simulink model "amisa"  (R2013a)
settings: Solver=VariableStepDiscrete  SolverMode=SingleTasking  StartTime=0.0  StopTime=5000  RelTol=1e-3
undefined symbols (not defined in the file or in its folder): gcbh, sfp, xlBlockLoadCallback
libraries: xbsIndex_r4 x4683, dspsigops x32, xps_library x30, casper_library_misc x27, casper_library_delays x2
(part 8 of 43)

== system amisa/gpio_switch_states ==
  addr : Inport
  data_in : Inport  Port=2
  we : Inport  Port=3
  amisa_gpio_switch_states_addr : xbsIndex_r4/Gateway Out  inherit_from_input=off  hdl_port=on  timing_constraint=None  locs_specified=off  LOCs={'A5','B9','A9','C1','A3','G6','E9','A6','A7','A8','B8','B1','B3','D9','B5','B4','B6','C2'}  UseAsDAC=off  DACChannel='1'  block_type=gatewayout
      settings: infoedit="Gateway out block.  Converts Xilinx fixed point inputs into ouputs of type Simulink integer, double, or fixed point.<P><P>Hardware notes:  In hardware these blocks become top level output ports or are discarded, depending on how they are configured."  xl_area=[0, 0, 0, 0, 0, 0, 0]  sginterface={'Nallatech'=>{'xdspkit'=>{'non_memory_mapped_port'=>'uprev_Shared_BRAM_addr'}},'Xilinx'=>{'jtaghwcosim'=>{'non_memory_mapped_port'=>'uprev_Shared_BRAM_addr'},'xdspkit'=>{'non_memory_mapped_port'=>'uprev_Shared_BRAM_addr'}}}
  amisa_gpio_switch_states_data_in : xbsIndex_r4/Gateway Out  inherit_from_input=off  hdl_port=on  timing_constraint=None  locs_specified=off  LOCs={'B21','B22','A22','B23','B19','C19','A20','A21','A23','B24','A24','A25','E18','D18','C18','B18'}  UseAsDAC=off  DACChannel='1'  block_type=gatewayout
      settings: infoedit="Gateway out block.  Converts Xilinx fixed point inputs into ouputs of type Simulink integer, double, or fixed point.<P><P>Hardware notes:  In hardware these blocks become top level output ports or are discarded, depending on how they are configured."  xl_area=[0, 0, 0, 0, 0, 0, 0]  sginterface={'Nallatech'=>{'xdspkit'=>{'non_memory_mapped_port'=>'uprev_Shared_BRAM_data_in'}},'Xilinx'=>{'jtaghwcosim'=>{'non_memory_mapped_port'=>'uprev_Shared_BRAM_data_in'},'xdspkit'=>{'non_memory_mapped_port'=>'uprev_Shared_BRAM_data_in'}}}
  amisa_gpio_switch_states_data_out : xbsIndex_r4/Gateway In  gui_display_data_type=Fixed-point  arith_type=Unsigned  n_bits=8  bin_pt=0  preci_type=Single  exp_width=8  frac_width=24  quantization=Truncate  overflow=Wrap  period=sample_rate  dbl_ovrd=off  timing_constraint=None  locs_specified=off  LOCs={}  UseAsADC=off  ADCChannel='1'  inherit_from_input=off  hdl_port=on  block_type=gatewayin
      settings: xl_area=[0, 0, 0, 0, 0, 0, 0]
  amisa_gpio_switch_states_we : xbsIndex_r4/Gateway Out  inherit_from_input=off  hdl_port=on  timing_constraint=None  locs_specified=off  LOCs={'A14'}  UseAsDAC=off  DACChannel='1'  block_type=gatewayout
      settings: infoedit="Gateway out block.  Converts Xilinx fixed point inputs into ouputs of type Simulink integer, double, or fixed point.<P><P>Hardware notes:  In hardware these blocks become top level output ports or are discarded, depending on how they are configured."  xl_area=[0, 0, 0, 0, 0, 0, 0]
  calc_add : Subsystem  mask{data_width=8, addr_width=12, sample_rate=sample_rate}
      mask prompts: data_width "data width"; addr_width "address width"; sample_rate "sample rate"
  convert_addr : xbsIndex_r4/Convert  gui_display_data_type=Fixed-point  arith_type=Unsigned  n_bits=addr_width  bin_pt=0  float_type=Single  exp_bits=8  fraction_bits=24  quantization=Truncate  overflow=Wrap  en=off  latency=0  dbl_ovrd=off  pipeline=off  block_type=convert
      settings: xl_area=[0, 0, 0, 0, 0, 0, 0]
  convert_din1 : xbsIndex_r4/Convert  gui_display_data_type=Fixed-point  arith_type=Unsigned  n_bits=8  bin_pt=0  float_type=Single  exp_bits=8  fraction_bits=24  quantization=Truncate  overflow=Wrap  en=off  latency=0  dbl_ovrd=off  pipeline=off  block_type=convert
      settings: xl_area=[0, 0, 0, 0, 0, 0, 0]
  convert_we : xbsIndex_r4/Convert  gui_display_data_type=Fixed-point  arith_type=Unsigned  n_bits=1  bin_pt=0  float_type=Single  exp_bits=8  fraction_bits=24  quantization=Truncate  overflow=Wrap  en=off  latency=0  dbl_ovrd=off  pipeline=off  block_type=convert
      settings: xl_area=[0, 0, 0, 0, 0, 0, 0]
  mem : Subsystem
  munge_in : Subsystem  AncestorBlock=casper_library_flow_control/munge  mask(munge){divisions=1, div_size=8, order=[0], arith_type_out=Unsigned, bin_pt_out=0}
      mask prompts: divisions "Number of divisions"; div_size "Division size (bits)"; order "Division packing order"; arith_type_out "Output arithmetic type"; bin_pt_out "Output binary point"
      mask help: Splits an input bus into the specified number of divisions and then recombines them in the order specified (most significant division = 0,least = number divisions-1)
      mask init:
      | munge_init(gcb, ...
      |     'divisions', divisions, ...
      |     'div_size', div_size, ...
      |     'order', order, ...
      |     'arith_type_out', arith_type_out, ...
      |     'bin_pt_out', bin_pt_out);
      settings: AttributesFormatString=|
      | split:8
      | join:0
      | Unsigned [8,0]
      mask TypeOptions arith_type_out: Unsigned | Signed  (2's comp) | Floating-point
  munge_out : Subsystem  AncestorBlock=casper_library_flow_control/munge  mask(munge){divisions=1, div_size=8, order=[0], arith_type_out=Unsigned, bin_pt_out=0}
      mask prompts: divisions "Number of divisions"; div_size "Division size (bits)"; order "Division packing order"; arith_type_out "Output arithmetic type"; bin_pt_out "Output binary point"
      mask help: Splits an input bus into the specified number of divisions and then recombines them in the order specified (most significant division = 0,least = number divisions-1)
      mask init:
      | munge_init(gcb, ...
      |     'divisions', divisions, ...
      |     'div_size', div_size, ...
      |     'order', order, ...
      |     'arith_type_out', arith_type_out, ...
      |     'bin_pt_out', bin_pt_out);
      settings: AttributesFormatString=|
      | split:8
      | join:0
      | Unsigned [8,0]
      mask TypeOptions arith_type_out: Unsigned | Signed  (2's comp) | Floating-point
  data_out : Outport
  wires:
  convert_addr/1 -> amisa_gpio_switch_states_addr/1
  convert_din1/1 -> amisa_gpio_switch_states_data_in/1
  data_in/1 -> munge_in/1(din)
  calc_add/1(out) -> convert_addr/1
  amisa_gpio_switch_states_we/1 -> mem/3(In3)
  amisa_gpio_switch_states_data_in/1 -> mem/2(In2)
  amisa_gpio_switch_states_addr/1 -> mem/1(In1)
  convert_we/1 -> amisa_gpio_switch_states_we/1
  amisa_gpio_switch_states_data_out/1 -> munge_out/1(din)
  mem/1(Out1) -> amisa_gpio_switch_states_data_out/1
  addr/1 -> calc_add/1(in)
  we/1 -> convert_we/1
  munge_out/1(dout) -> data_out/1
  munge_in/1(dout) -> convert_din1/1

== system amisa/ip_base ==
  sim_1 : Inport
  amisa_ip_base_user_data_out : xbsIndex_r4/Gateway In  gui_display_data_type=Fixed-point  arith_type=Unsigned  n_bits=32  bin_pt=0  preci_type=Single  exp_width=8  frac_width=24  quantization="Round  (unbiased: +/- Inf)"  overflow=Saturate  period=1  dbl_ovrd=off  timing_constraint=None  locs_specified=off  LOCs={}  UseAsADC=off  ADCChannel='1'  inherit_from_input=off  hdl_port=on  block_type=gatewayin
  io_delay : xbsIndex_r4/Delay  rst=off  infoeditControl=Selection of Reset will increase slice count due to use of real FFs and instead of SRLs  en=off  latency=0  dbl_ovrd=off  reg_retiming=on  block_type=delay
  reint1 : xbsIndex_r4/Reinterpret  force_arith_type=on  arith_type=Unsigned  force_bin_pt=on  bin_pt=0  block_type=reinterpret
  slice_reg : xbsIndex_r4/Slice  nbits=32  boolean_output=off  mode=Lower Bit Location + Width  bit1=0  base1=MSB of Input  bit0=0  base0=LSB of Input  dbl_ovrd=off  block_type=slice
  in_reg : Outport
  wires:
  amisa_ip_base_user_data_out/1 -> io_delay/1
  sim_1/1 -> amisa_ip_base_user_data_out/1
  io_delay/1 -> slice_reg/1
  slice_reg/1 -> reint1/1
  reint1/1 -> in_reg/1

== system amisa/leds ==
  warning : Inport
  rst : Inport  Port=2
  sync_led : Inport  Port=3
  pps : Inport  Port=4
  comms : Inport  Port=5
  ps_gpio : Inport  Port=6
  noise_gpio : Inport  Port=7
  or0 : Inport  Port=8
  or1 : Inport  Port=9
  0 : xps_library/gpio  Tag=xps:gpio  io_group=ROACH2:led  io_dir=out  arith_type=Boolean  bitwidth=1  bin_pt=0  bit_index=0  sample_period=1  use_single_ended=off  use_ddr=off  reg_iob=on  reg_clk_phase=0  termination=None
      link override convert: arith_type=Boolean  n_bits=1  bin_pt=0
  1 : xps_library/gpio  Tag=xps:gpio  io_group=ROACH2:led  io_dir=out  arith_type=Boolean  bitwidth=1  bin_pt=0  bit_index=1  sample_period=1  use_single_ended=off  use_ddr=off  reg_iob=on  reg_clk_phase=0  termination=None
      link override convert: arith_type=Boolean  n_bits=1  bin_pt=0
  2 : xps_library/gpio  Tag=xps:gpio  io_group=ROACH2:led  io_dir=out  arith_type=Boolean  bitwidth=1  bin_pt=0  bit_index=2  sample_period=1  use_single_ended=off  use_ddr=off  reg_iob=on  reg_clk_phase=0  termination=None
      link override convert: arith_type=Boolean  n_bits=1  bin_pt=0
  3 : xps_library/gpio  Tag=xps:gpio  io_group=ROACH2:led  io_dir=out  arith_type=Boolean  bitwidth=1  bin_pt=0  bit_index=3  sample_period=1  use_single_ended=off  use_ddr=off  reg_iob=on  reg_clk_phase=0  termination=None
      link override convert: arith_type=Boolean  n_bits=1  bin_pt=0
  4 : xps_library/gpio  Tag=xps:gpio  io_group=ROACH2:led  io_dir=out  arith_type=Boolean  bitwidth=1  bin_pt=0  bit_index=4  sample_period=1  use_single_ended=off  use_ddr=off  reg_iob=on  reg_clk_phase=0  termination=None
      link override convert: arith_type=Boolean  n_bits=1  bin_pt=0
  5 : xps_library/gpio  Tag=xps:gpio  io_group=ROACH2:led  io_dir=out  arith_type=Boolean  bitwidth=1  bin_pt=0  bit_index=5  sample_period=1  use_single_ended=off  use_ddr=off  reg_iob=on  reg_clk_phase=0  termination=None
      link override convert: arith_type=Boolean  n_bits=1  bin_pt=0
  6 : xps_library/gpio  Tag=xps:gpio  io_group=ROACH2:led  io_dir=out  arith_type=Boolean  bitwidth=1  bin_pt=0  bit_index=6  sample_period=1  use_single_ended=off  use_ddr=off  reg_iob=on  reg_clk_phase=0  termination=None
      link override convert: arith_type=Boolean  n_bits=1  bin_pt=0
  7 : xps_library/gpio  Tag=xps:gpio  io_group=ROACH2:led  io_dir=out  arith_type=Boolean  bitwidth=1  bin_pt=0  bit_index=7  sample_period=1  use_single_ended=off  use_ddr=off  reg_iob=on  reg_clk_phase=0  termination=None
      link override convert: arith_type=Boolean  n_bits=1  bin_pt=0
  Counter1 : xbsIndex_r4/Counter  cnt_type=Free Running  cnt_to=Inf  operation=Up  start_count=0  cnt_by_val=1  arith_type=Unsigned  n_bits=1  bin_pt=0  load_pin=off  rst=on  en=on  explicit_period=on  period=1  dbl_ovrd=off  use_behavioral_HDL=off  implementation=Fabric  use_rpm=off  block_type=counter
  Counter2 : xbsIndex_r4/Counter  cnt_type=Free Running  cnt_to=Inf  operation=Up  start_count=0  cnt_by_val=1  arith_type=Unsigned  n_bits=1  bin_pt=0  load_pin=off  rst=on  en=on  explicit_period=on  period=1  dbl_ovrd=off  use_behavioral_HDL=off  implementation=Fabric  use_rpm=off  block_type=counter
  Logical2 : xbsIndex_r4/Logical  logical_function=OR  inputs=3  en=off  latency=1  precision=Full  arith_type=Unsigned  n_bits=16  bin_pt=0  align_bp=on  dbl_ovrd=off  block_type=logical
      settings: block_version=11.4
  Logical{3..6} (4 alike) : xbsIndex_r4/Logical  logical_function=OR  inputs=2  en=off  latency=1  precision=Full  arith_type=Unsigned  n_bits=16  bin_pt=0  align_bp=on  dbl_ovrd=off  block_type=logical
      settings: block_version=11.4
  Slice{,1..3} (4 alike) : xbsIndex_r4/Slice  nbits=1  boolean_output=on  mode=Upper Bit Location + Width  bit1=0  base1=MSB of Input  bit0=0  base0=LSB of Input  dbl_ovrd=off  block_type=slice
  Terminator{5..8,10..13} (8 alike) : Terminator
  pipeline : Subsystem  AncestorBlock=casper_library_delays/pipeline  mask(pipeline){latency=3}
      mask help:
      | An explicitly laid-out delay line to avoid mapping to SRL16s
      | for use in pipelining to help achieve timing closure.
      mask init:
      | pipeline_init(gcb,'latency',latency);
      settings: AttributesFormatString=Latency = %<latency>
      mask Display:
      | port_label('input', 1, 'd');
      | port_label('output', 1, 'q');
      | disp(['Z^-', num2str(latency)]);
  pipeline1 : Subsystem  AncestorBlock=casper_library_delays/pipeline  mask(pipeline){latency=3}
      mask help:
      | An explicitly laid-out delay line to avoid mapping to SRL16s
      | for use in pipelining to help achieve timing closure.
      mask init:
      | pipeline_init(gcb,'latency',latency);
      settings: AttributesFormatString=Latency = %<latency>
      mask Display:
      | port_label('input', 1, 'd');
      | port_label('output', 1, 'q');
      | disp(['Z^-', num2str(latency)]);
  pipeline12 : Subsystem  AncestorBlock=casper_library_delays/pipeline  mask(pipeline){latency=2}
      mask help:
      | An explicitly laid-out delay line to avoid mapping to SRL16s
      | for use in pipelining to help achieve timing closure.
      mask init:
      | pipeline_init(gcb,'latency',latency);
      settings: AttributesFormatString=Latency = %<latency>
      mask Display:
      | port_label('input', 1, 'd');
      | port_label('output', 1, 'q');
      | disp(['Z^-', num2str(latency)]);
  pipeline13 : Subsystem  AncestorBlock=casper_library_delays/pipeline  mask(pipeline){latency=2}
      mask help:
      | An explicitly laid-out delay line to avoid mapping to SRL16s
      | for use in pipelining to help achieve timing closure.
      mask init:
      | pipeline_init(gcb,'latency',latency);
      settings: AttributesFormatString=Latency = %<latency>
      mask Display:
      | port_label('input', 1, 'd');
      | port_label('output', 1, 'q');
      | disp(['Z^-', num2str(latency)]);
  pipeline14 : Subsystem  AncestorBlock=casper_library_delays/pipeline  mask(pipeline){latency=2}
      mask help:
      | An explicitly laid-out delay line to avoid mapping to SRL16s
      | for use in pipelining to help achieve timing closure.
      mask init:
      | pipeline_init(gcb,'latency',latency);
      settings: AttributesFormatString=Latency = %<latency>
      mask Display:
      | port_label('input', 1, 'd');
      | port_label('output', 1, 'q');
      | disp(['Z^-', num2str(latency)]);
  pipeline2 : Subsystem  AncestorBlock=casper_library_delays/pipeline  mask(pipeline){latency=3}
      mask help:
      | An explicitly laid-out delay line to avoid mapping to SRL16s
      | for use in pipelining to help achieve timing closure.
      mask init:
      | pipeline_init(gcb,'latency',latency);
      settings: AttributesFormatString=Latency = %<latency>
      mask Display:
      | port_label('input', 1, 'd');
      | port_label('output', 1, 'q');
      | disp(['Z^-', num2str(latency)]);
  pipeline3 : Subsystem  AncestorBlock=casper_library_delays/pipeline  mask(pipeline){latency=3}
      mask help:
      | An explicitly laid-out delay line to avoid mapping to SRL16s
      | for use in pipelining to help achieve timing closure.
      mask init:
      | pipeline_init(gcb,'latency',latency);
      settings: AttributesFormatString=Latency = %<latency>
      mask Display:
      | port_label('input', 1, 'd');
      | port_label('output', 1, 'q');
      | disp(['Z^-', num2str(latency)]);
  pipeline4 : Subsystem  AncestorBlock=casper_library_delays/pipeline  mask(pipeline){latency=3}
      mask help:
      | An explicitly laid-out delay line to avoid mapping to SRL16s
      | for use in pipelining to help achieve timing closure.
      mask init:
      | pipeline_init(gcb,'latency',latency);
      settings: AttributesFormatString=Latency = %<latency>
      mask Display:
      | port_label('input', 1, 'd');
      | port_label('output', 1, 'q');
      | disp(['Z^-', num2str(latency)]);
  pipeline5 : Subsystem  AncestorBlock=casper_library_delays/pipeline  mask(pipeline){latency=3}
      mask help:
      | An explicitly laid-out delay line to avoid mapping to SRL16s
      | for use in pipelining to help achieve timing closure.
      mask init:
      | pipeline_init(gcb,'latency',latency);
      settings: AttributesFormatString=Latency = %<latency>
      mask Display:
      | port_label('input', 1, 'd');
      | port_label('output', 1, 'q');
      | disp(['Z^-', num2str(latency)]);
  pipeline6 : Subsystem  AncestorBlock=casper_library_delays/pipeline  mask(pipeline){latency=3}
      mask help:
      | An explicitly laid-out delay line to avoid mapping to SRL16s
      | for use in pipelining to help achieve timing closure.
      mask init:
      | pipeline_init(gcb,'latency',latency);
      settings: AttributesFormatString=Latency = %<latency>
      mask Display:
      | port_label('input', 1, 'd');
      | port_label('output', 1, 'q');
      | disp(['Z^-', num2str(latency)]);
  pipeline7 : Subsystem  AncestorBlock=casper_library_delays/pipeline  mask(pipeline){latency=3}
      mask help:
      | An explicitly laid-out delay line to avoid mapping to SRL16s
      | for use in pipelining to help achieve timing closure.
      mask init:
      | pipeline_init(gcb,'latency',latency);
      settings: AttributesFormatString=Latency = %<latency>
      mask Display:
      | port_label('input', 1, 'd');
      | port_label('output', 1, 'q');
      | disp(['Z^-', num2str(latency)]);
  pipeline8 : Subsystem  AncestorBlock=casper_library_delays/pipeline  mask(pipeline){latency=2}
      mask help:
      | An explicitly laid-out delay line to avoid mapping to SRL16s
      | for use in pipelining to help achieve timing closure.
      mask init:
      | pipeline_init(gcb,'latency',latency);
      settings: AttributesFormatString=Latency = %<latency>
      mask Display:
      | port_label('input', 1, 'd');
      | port_label('output', 1, 'q');
      | disp(['Z^-', num2str(latency)]);
  pulse_ext{,1..3} (4 alike) : casper_library_misc/pulse_ext  pulse_len=2^24
  pulse_ext4 : casper_library_misc/pulse_ext  pulse_len=2^21
  pulse_ext5 : casper_library_misc/pulse_ext  pulse_len=2^21
  wires:
  0/1 -> Terminator5/1
  1/1 -> Terminator6/1
  4/1 -> Terminator7/1
  5/1 -> Terminator8/1
  6/1 -> Terminator10/1
  7/1 -> Terminator11/1
  pipeline6/1(q) -> 2/1
  pipeline7/1(q) -> 3/1
  comms/1 -> pulse_ext3/1
  warning/1 -> [warning]
  [comms] -> Slice3/1
  [warning_led] -> Slice2/1
  Slice2/1 -> pipeline1/1(d)
  [or1] -> pipeline2/1(d)
  [or0] -> pipeline3/1(d)
  [pps] -> Slice/1
  Logical6/1 -> pipeline4/1(d)
  Logical5/1 -> pipeline5/1(d)
  [sync] -> Slice1/1
  Logical4/1 -> pipeline6/1(d)
  Logical3/1 -> pipeline7/1(d)
  or0/1 -> pulse_ext/1
  or1/1 -> pulse_ext1/1
  pulse_ext/1 -> pipeline13/1(d)
  pulse_ext1/1 -> pipeline14/1(d)
  rst/1 -> pulse_ext2/1
  pps/1 -> Counter2/2
  sync_led/1 -> Counter1/2
  [rst] -> Counter2/1
  [rst] -> Counter1/1
  ps_gpio/1 -> pulse_ext5/1
  noise_gpio/1 -> pulse_ext4/1
  pulse_ext3/1 -> pipeline12/1(d)
  [warning] -> Logical2/1
  [or0] -> Logical2/2
  [or1] -> Logical2/3
  Logical2/1 -> [warning_led]
  Counter2/1 -> [pps]
  Counter1/1 -> [sync]
  pipeline/1(q) -> 4/1
  pipeline1/1(q) -> 5/1
  pipeline2/1(q) -> 6/1
  pipeline3/1(q) -> 7/1
  pipeline4/1(q) -> 0/1
  pipeline5/1(q) -> 1/1
  pipeline12/1(q) -> [comms]
  pipeline13/1(q) -> [or0]
  pipeline14/1(q) -> [or1]
  2/1 -> Terminator12/1
  3/1 -> Terminator13/1
  Slice/1 -> Logical6/1
  Slice1/1 -> Logical5/1
  [noise_gpio] -> Logical4/1
  [ps_gpio] -> Logical3/1
  pulse_ext2/1 -> pipeline8/1(d)
  pipeline8/1(q) -> [rst]
  [rst] -> Logical6/2, Logical5/2, Logical4/2, Logical3/2
  Slice3/1 -> pipeline/1(d)
  pulse_ext4/1 -> [noise_gpio]
  pulse_ext5/1 -> [ps_gpio]

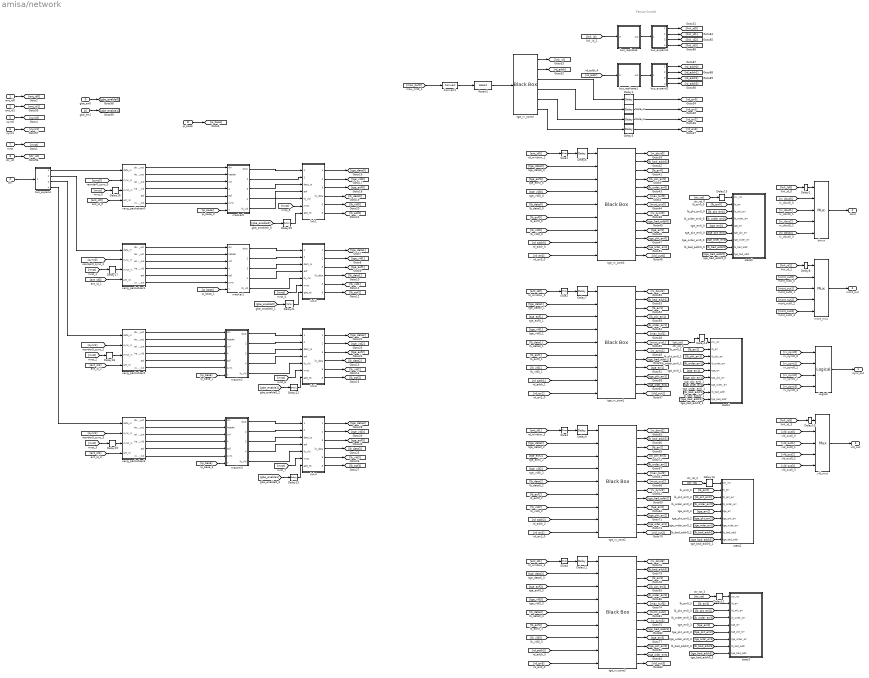
== system amisa/network ==
  note: Fanout Control
  ant_id0 : Inport
  ant_id1 : Inport  Port=2
  ctr_rst : Inport  Port=3
  din : Inport  Port=4
  sync0 : Inport  Port=5
  sync1 : Inport  Port=6
  mrst : Inport  Port=7
  ip_base : Inport  Port=8
  gbe_en0 : Inport  Port=9
  gbe_en1 : Inport  Port=10
  Assert1 : xbsIndex_r4/Assert  assert_type=off  type_source=Explicitly  gui_display_data_type=Fixed-point  arith_type="Signed  (2's comp)"  n_bits=16  bin_pt=14  preci_type=Single  exp_width=8  frac_width=24  assert_rate=on  rate_source=Explicitly  period=1  output_port=on  block_type=assert
  Convert1 : xbsIndex_r4/Convert  gui_display_data_type=Fixed-point  arith_type=Unsigned  n_bits=7  bin_pt=0  float_type=Single  exp_bits=8  fraction_bits=24  quantization=Truncate  overflow=Wrap  en=off  latency=0  dbl_ovrd=off  pipeline=off  block_type=convert
      settings: block_version=11.4
  Delay{1,3..5} (4 alike) : xbsIndex_r4/Delay  rst=off  infoeditControl=Selection of Reset will increase slice count due to use of real FFs and instead of SRLs  en=off  latency=2  dbl_ovrd=off  reg_retiming=on  block_type=delay
  Delay10 : xbsIndex_r4/Delay  rst=off  infoeditControl=Selection of Reset will increase slice count due to use of real FFs and instead of SRLs  en=off  latency=8  dbl_ovrd=off  reg_retiming=on  block_type=delay
  Delay{6..7,9,11..23} (16 alike) : xbsIndex_r4/Delay  rst=off  infoeditControl=Selection of Reset will increase slice count due to use of real FFs and instead of SRLs  en=off  latency=1  dbl_ovrd=off  reg_retiming=off  block_type=delay
  Delay2 : xbsIndex_r4/Delay  rst=off  infoeditControl=Selection of Reset will increase slice count due to use of real FFs and instead of SRLs  en=off  latency=8  dbl_ovrd=off  reg_retiming=on  block_type=delay
  Delay8 : xbsIndex_r4/Delay  rst=off  infoeditControl=Selection of Reset will increase slice count due to use of real FFs and instead of SRLs  en=off  latency=8  dbl_ovrd=off  reg_retiming=on  block_type=delay
  Logical : xbsIndex_r4/Logical  logical_function=OR  inputs=4  en=off  latency=1  precision=Full  arith_type=Unsigned  n_bits=16  bin_pt=0  align_bp=on  dbl_ovrd=off  block_type=logical
  Slice{1..4} (4 alike) : xbsIndex_r4/Slice  nbits=4  boolean_output=off  mode=Lower Bit Location + Width  bit1=0  base1=MSB of Input  bit0=0  base0=LSB of Input  dbl_ovrd=off  block_type=slice
  bus_expand : Subsystem  AncestorBlock=casper_library_flow_control/bus_expand  mask(bus_expand){mode=divisions of equal size, outputNum=4, outputWidth=32, outputBinaryPt=0, outputArithmeticType=0, show_format=off, outputToWorkspace=off, variablePrefix=out, outputToModelAsWell=on}
      mask prompts: outputNum "Number of outputs:"; outputWidth "Output width:"; outputBinaryPt "Output binary point position:"; outputArithmeticType "Output arithmetic type (ufix=0, fix=1, bool=2):"; show_format "Print format string?"; outputToWorkspace "Output to workspace?"; variablePrefix "Variable name prefix:"; outputToModelAsWell "Output to model as well?"
      mask help:
      | Expands a 'bus' made using a bus_create or Xilinx
      | concat block.
      | The input will be divided into the specified number
      | of outputs with the specified arithmetic types.
      | Divisions are made from most significant bit.
      mask init: same as amisa/bus_expand6
      settings: AttributesFormatString=4 outputs
      mask TypeOptions mode: divisions of equal size | divisions of arbitrary size
      mask Callback mode: bus_expand_callback();
      mask Callback outputWidth: bus_expand_callback();
      mask Callback outputToWorkspace: bus_expand_callback();
  bus_expand1 : Subsystem  AncestorBlock=casper_library_flow_control/bus_expand  mask(bus_expand){mode=divisions of equal size, outputNum=4, outputWidth=2, outputBinaryPt=0, outputArithmeticType=0, show_format=off, outputToWorkspace=off, variablePrefix=out, outputToModelAsWell=on}
      mask prompts: outputNum "Number of outputs:"; outputWidth "Output width:"; outputBinaryPt "Output binary point position:"; outputArithmeticType "Output arithmetic type (ufix=0, fix=1, bool=2):"; show_format "Print format string?"; outputToWorkspace "Output to workspace?"; variablePrefix "Variable name prefix:"; outputToModelAsWell "Output to model as well?"
      mask help:
      | Expands a 'bus' made using a bus_create or Xilinx
      | concat block.
      | The input will be divided into the specified number
      | of outputs with the specified arithmetic types.
      | Divisions are made from most significant bit.
      mask init: same as amisa/bus_expand6
      settings: AttributesFormatString=4 outputs
      mask TypeOptions mode: divisions of equal size | divisions of arbitrary size
      mask Callback mode: bus_expand_callback();
      mask Callback outputWidth: bus_expand_callback();
      mask Callback outputToWorkspace: bus_expand_callback();
  bus_expand2 : Subsystem  AncestorBlock=casper_library_flow_control/bus_expand  mask(bus_expand){mode=divisions of equal size, outputNum=4, outputWidth=13, outputBinaryPt=0, outputArithmeticType=0, show_format=off, outputToWorkspace=off, variablePrefix=out, outputToModelAsWell=on}
      mask prompts: outputNum "Number of outputs:"; outputWidth "Output width:"; outputBinaryPt "Output binary point position:"; outputArithmeticType "Output arithmetic type (ufix=0, fix=1, bool=2):"; show_format "Print format string?"; outputToWorkspace "Output to workspace?"; variablePrefix "Variable name prefix:"; outputToModelAsWell "Output to model as well?"
      mask help:
      | Expands a 'bus' made using a bus_create or Xilinx
      | concat block.
      | The input will be divided into the specified number
      | of outputs with the specified arithmetic types.
      | Divisions are made from most significant bit.
      mask init: same as amisa/bus_expand6
      settings: AttributesFormatString=4 outputs
      mask TypeOptions mode: divisions of equal size | divisions of arbitrary size
      mask Callback mode: bus_expand_callback();
      mask Callback outputWidth: bus_expand_callback();
      mask Callback outputToWorkspace: bus_expand_callback();
  bus_replicate : Subsystem  AncestorBlock=casper_library_bus/bus_replicate  mask(bus_replicate){replication=4, latency=2, misc=off, implementation=core}
      mask prompts: replication "replication factor"; misc "misc support"; implementation "delay implementation"
      mask help: Output bus formed by replicating input bus a number of times
      mask init:
      | bus_replicate_init(gcb, ...
      |     'replication', replication, ...
      |     'latency', latency, ...
      |     'implementation', implementation, ...
      |     'misc', misc);
      mask TypeOptions implementation: core | behavioral
  bus_replicate1 : Subsystem  AncestorBlock=casper_library_bus/bus_replicate  mask(bus_replicate){replication=4, latency=2, misc=off, implementation=core}
      mask prompts: replication "replication factor"; misc "misc support"; implementation "delay implementation"
      mask help: Output bus formed by replicating input bus a number of times
      mask init:
      | bus_replicate_init(gcb, ...
      |     'replication', replication, ...
      |     'latency', latency, ...
      |     'implementation', implementation, ...
      |     'misc', misc);
      mask TypeOptions implementation: core | behavioral
  dmux : xbsIndex_r4/Mux  inputs=4  en=off  latency=1  precision=Full  arith_type=Unsigned  n_bits=16  bin_pt=14  quantization=Truncate  overflow=Wrap  dbl_ovrd=off  block_type=mux
  link1 : Subsystem
  link2 : Subsystem
  link3 : Subsystem
  link4 : Subsystem
  masker0 : Subsystem  mask{n_chan_bits=10}
      mask prompts: n_chan_bits "Number of channels on this link (2^?)"
  masker1 : Subsystem  mask{n_chan_bits=10}
      mask prompts: n_chan_bits "Number of channels on this link (2^?)"
  masker2 : Subsystem  mask{n_chan_bits=10}
      mask prompts: n_chan_bits "Number of channels on this link (2^?)"
  masker3 : Subsystem  mask{n_chan_bits=10}
      mask prompts: n_chan_bits "Number of channels on this link (2^?)"
  mcnt_mux : xbsIndex_r4/Mux  inputs=4  en=off  latency=1  precision=Full  arith_type=Unsigned  n_bits=16  bin_pt=14  quantization=Truncate  overflow=Wrap  dbl_ovrd=off  block_type=mux
  stats0 : Subsystem
  stats1 : Subsystem
  stats2 : Subsystem
  stats3 : Subsystem
  tge_rx_core{0..3} (4 alike) : xbsIndex_r4/Black Box  init_code=tge_rx_core_config  sim_method=Inactive  verbose=off  block_type=blackbox2
  tge_rx_core4 : xbsIndex_r4/Black Box  init_code=tge_rx_out_core_config  sim_method=Inactive  verbose=off  block_type=blackbox2
  vld_mux : xbsIndex_r4/Mux  inputs=4  en=off  latency=1  precision=Full  arith_type=Unsigned  n_bits=16  bin_pt=14  quantization=Truncate  overflow=Wrap  dbl_ovrd=off  block_type=mux
  xeng_packetiser0 : Subsystem  mask{nwrd_bits=10-3, n_packetizer_bits=1, chan_id=0, nband_bits=1, nchan_bits=10, band_id=0}
      mask prompts: nwrd_bits "Payload length: (in 64bit words) (2^n)"; n_packetizer_bits "Number of output streams (2^n)"; chan_id "Output stream (i.e. channel) id"; nband_bits "Number of bands (2^?)"; nchan_bits "Number of channels per output link (2^?)"; band_id "This band id?"
      mask help: Package 32 bit data into 64 bits and identify data as coming from antenna 0 or 1
  xeng_packetiser1 : Subsystem  mask{nwrd_bits=10-3, n_packetizer_bits=1, chan_id=1, nband_bits=1, nchan_bits=10, band_id=0}
      mask prompts: nwrd_bits "Payload length: (in 64bit words) (2^n)"; n_packetizer_bits "Number of output streams (2^n)"; chan_id "Output stream (i.e. channel) id"; nband_bits "Number of bands (2^?)"; nchan_bits "Number of channels per output link (2^?)"; band_id "This band id?"
      mask help: Package 32 bit data into 64 bits and identify data as coming from antenna 0 or 1
  xeng_packetiser2 : Subsystem  mask{nwrd_bits=10-3, n_packetizer_bits=1, chan_id=0, nband_bits=1, nchan_bits=10, band_id=1}
      mask prompts: nwrd_bits "Payload length: (in 64bit words) (2^n)"; n_packetizer_bits "Number of output streams (2^n)"; chan_id "Output stream (i.e. channel) id"; nband_bits "Number of bands (2^?)"; nchan_bits "Number of channels per output link (2^?)"; band_id "This band id?"
      mask help: Package 32 bit data into 64 bits and identify data as coming from antenna 0 or 1
  xeng_packetiser3 : Subsystem  mask{nwrd_bits=10-3, n_packetizer_bits=1, chan_id=1, nband_bits=1, nchan_bits=10, band_id=1}
      mask prompts: nwrd_bits "Payload length: (in 64bit words) (2^n)"; n_packetizer_bits "Number of output streams (2^n)"; chan_id "Output stream (i.e. channel) id"; nband_bits "Number of bands (2^?)"; nchan_bits "Number of channels per output link (2^?)"; band_id "This band id?"
      mask help: Package 32 bit data into 64 bits and identify data as coming from antenna 0 or 1
  sync_out : Outport
  dout : Outport  Port=2
  vld_out : Outport  Port=3
  mcnt_out : Outport  Port=4
  wires:
  [mrst] -> Delay16/1
  [sync0] -> xeng_packetiser1/2(sync_in)
  [mrst] -> Delay17/1
  [mrst] -> Delay18/1
  [sync1] -> xeng_packetiser3/2(sync_in)
  [mrst] -> Delay19/1
  [sync1] -> xeng_packetiser2/2(sync_in)
  bus_expand/4(lsb_out1) -> xeng_packetiser3/1(data_in)
  bus_expand/3(out2) -> xeng_packetiser2/1(data_in)
  din/1 -> bus_expand/1(bus_in)
  bus_expand/1(msb_out4) -> xeng_packetiser0/1(data_in)
  [sync0] -> xeng_packetiser0/2(sync_in)
  bus_expand/2(out3) -> xeng_packetiser1/1(data_in)
  sync0/1 -> [sync0]
  mrst/1 -> [mrst]
  ant_id0/1 -> [ant_id0]
  [ant_id0] -> xeng_packetiser0/4(ant_id)
  [ant_id0] -> xeng_packetiser1/4(ant_id)
  [ant_id1] -> xeng_packetiser2/4(ant_id)
  [ant_id1] -> xeng_packetiser3/4(ant_id)
  ip_base/1 -> [ip_base]
  [ip_base] -> masker0/7(ip_base)
  masker0/1(dout) -> link1/1(tx_data)
  masker0/2(gbe_vld) -> link1/2(gbe_vld)
  masker0/3(ip_addr) -> link1/3(dest_ip)
  masker0/4(eof_out) -> link1/4(eof)
  masker0/5(lb_vld) -> link1/5(lb_vld)
  [mrst] -> link1/6(mrst)
  link1/1(gbe_data) -> [tge_data0]
  link1/2(gbe_vld_out) -> [tge_vld0]
  link1/3(gbe_eof_out) -> [tge_eof0]
  link1/6(lb_eof_out) -> [lb_eof0]
  link1/4(lb_data) -> [lb_data0]
  link1/5(lb_vld_out) -> [lb_vld0]
  link2/1(gbe_data) -> [tge_data1]
  link2/2(gbe_vld_out) -> [tge_vld1]
  link2/3(gbe_eof_out) -> [tge_eof1]
  link2/6(lb_eof_out) -> [lb_eof1]
  link2/4(lb_data) -> [lb_data1]
  link2/5(lb_vld_out) -> [lb_vld1]
  link3/1(gbe_data) -> [tge_data2]
  link3/2(gbe_vld_out) -> [tge_vld2]
  link3/3(gbe_eof_out) -> [tge_eof2]
  link3/6(lb_eof_out) -> [lb_eof2]
  link3/4(lb_data) -> [lb_data2]
  link3/5(lb_vld_out) -> [lb_vld2]
  link4/1(gbe_data) -> [tge_data3]
  link4/2(gbe_vld_out) -> [tge_vld3]
  link4/3(gbe_eof_out) -> [tge_eof3]
  link4/6(lb_eof_out) -> [lb_eof3]
  link4/4(lb_data) -> [lb_data3]
  link4/5(lb_vld_out) -> [lb_vld3]
  tge_rx_core4/2 -> [rd_addr]
  tge_rx_core4/1 -> [link_id]
  tge_rx_core4/3 -> Delay1/1
  tge_rx_core4/5 -> Delay4/1
  tge_rx_core4/4 -> Delay3/1
  tge_rx_core4/6 -> Delay5/1
  [ant_id0] -> Slice1/1
  [rd_en0] -> tge_rx_core0/9
  [rd_addr0] -> tge_rx_core0/8
  [lb_vld0] -> tge_rx_core0/7
  [tge_eof0] -> tge_rx_core0/3
  [tge_data0] -> tge_rx_core0/2
  [lb_data0] -> tge_rx_core0/5
  [tge_vld0] -> tge_rx_core0/4
  [lb_eof0] -> tge_rx_core0/6
  tge_rx_core0/8 -> [rx_sync0]
  tge_rx_core0/1 -> [rx_dout0]
  tge_rx_core0/10 -> [tge_err0]
  tge_rx_core0/3 -> [lb_err0]
  tge_rx_core0/2 -> [lb_bad_addr0]
  tge_rx_core0/7 -> [mcnt_out0]
  tge_rx_core0/9 -> [tge_bad_addr0]
  [vld_out1] -> vld_mux/3
  [vld_out3] -> vld_mux/5
  [vld_out0] -> vld_mux/2
  [vld_out2] -> vld_mux/4
  [link_id3] -> Delay10/1
  [rx_sync3] -> Logical/4
  [rx_sync2] -> Logical/3
  [rx_sync1] -> Logical/2
  [rx_sync0] -> Logical/1
  [mcnt_out3] -> mcnt_mux/5
  [link_id1] -> Delay8/1
  [mcnt_out1] -> mcnt_mux/3
  [mcnt_out2] -> mcnt_mux/4
  [mcnt_out0] -> mcnt_mux/2
  [rx_dout2] -> dmux/4
  [rx_dout1] -> dmux/3
  [link_id0] -> Delay2/1
  [rx_dout3] -> dmux/5
  [rx_dout0] -> dmux/2
  dmux/1 -> dout/1
  vld_mux/1 -> vld_out/1
  Logical/1 -> sync_out/1
  mcnt_mux/1 -> mcnt_out/1
  Slice1/1 -> Delay6/1
  xeng_packetiser0/1(data_out) -> masker0/1(din)
  xeng_packetiser0/2(header_out) -> masker0/2(header)
  xeng_packetiser0/3(valid_out) -> masker0/3(vld)
  xeng_packetiser0/4(header_vld) -> masker0/4(header_vld)
  xeng_packetiser0/5(eof) -> masker0/5(eof)
  xeng_packetiser0/6(sync_out) -> masker0/6(sync)
  [ip_base] -> masker1/7(ip_base)
  xeng_packetiser1/1(data_out) -> masker1/1(din)
  xeng_packetiser1/2(header_out) -> masker1/2(header)
  xeng_packetiser1/3(valid_out) -> masker1/3(vld)
  xeng_packetiser1/4(header_vld) -> masker1/4(header_vld)
  xeng_packetiser1/5(eof) -> masker1/5(eof)
  xeng_packetiser1/6(sync_out) -> masker1/6(sync)
  [ip_base] -> masker2/7(ip_base)
  xeng_packetiser2/1(data_out) -> masker2/1(din)
  xeng_packetiser2/2(header_out) -> masker2/2(header)
  xeng_packetiser2/3(valid_out) -> masker2/3(vld)
  xeng_packetiser2/4(header_vld) -> masker2/4(header_vld)
  xeng_packetiser2/5(eof) -> masker2/5(eof)
  xeng_packetiser2/6(sync_out) -> masker2/6(sync)
  [ip_base] -> masker3/7(ip_base)
  xeng_packetiser3/1(data_out) -> masker3/1(din)
  xeng_packetiser3/2(header_out) -> masker3/2(header)
  xeng_packetiser3/3(valid_out) -> masker3/3(vld)
  xeng_packetiser3/4(header_vld) -> masker3/4(header_vld)
  xeng_packetiser3/5(eof) -> masker3/5(eof)
  xeng_packetiser3/6(sync_out) -> masker3/6(sync)
  tge_rx_core0/4 -> [lb_pkt_err0]
  tge_rx_core0/11 -> [tge_pkt_err0]
  [ant_id0] -> Slice2/1
  [rd_en1] -> tge_rx_core1/9
  [rd_addr1] -> tge_rx_core1/8
  [lb_vld1] -> tge_rx_core1/7
  [tge_eof1] -> tge_rx_core1/3
  [tge_data1] -> tge_rx_core1/2
  [lb_data1] -> tge_rx_core1/5
  [tge_vld1] -> tge_rx_core1/4
  [lb_eof1] -> tge_rx_core1/6
  Slice2/1 -> Delay7/1
  [ant_id1] -> Slice3/1
  [rd_en2] -> tge_rx_core2/9
  [rd_addr2] -> tge_rx_core2/8
  [lb_vld2] -> tge_rx_core2/7
  [tge_eof2] -> tge_rx_core2/3
  [tge_data2] -> tge_rx_core2/2
  [lb_data2] -> tge_rx_core2/5
  [tge_vld2] -> tge_rx_core2/4
  [lb_eof2] -> tge_rx_core2/6
  Slice3/1 -> Delay9/1
  [ant_id1] -> Slice4/1
  [rd_en3] -> tge_rx_core3/9
  [rd_addr3] -> tge_rx_core3/8
  [lb_vld3] -> tge_rx_core3/7
  [tge_eof3] -> tge_rx_core3/3
  [tge_data3] -> tge_rx_core3/2
  [lb_data3] -> tge_rx_core3/5
  [tge_vld3] -> tge_rx_core3/4
  [lb_eof3] -> tge_rx_core3/6
  Slice4/1 -> Delay11/1
  [max_buf0] -> Convert1/1
  Assert1/1 -> tge_rx_core4/1
  Delay2/1 -> dmux/1
  Delay8/1 -> mcnt_mux/1
  Delay10/1 -> vld_mux/1
  Convert1/1 -> Assert1/1
  bus_replicate/1(out) -> bus_expand1/1(bus_in)
  [link_id] -> bus_replicate/1(in)
  bus_replicate1/1(out) -> bus_expand2/1(bus_in)
  [rd_addr] -> bus_replicate1/1(in)
  bus_expand1/1(msb_out4) -> [link_id0]
  bus_expand1/3(out2) -> [link_id2]
  bus_expand1/4(lsb_out1) -> [link_id3]
  bus_expand1/2(out3) -> [link_id1]
  bus_expand2/4(lsb_out1) -> [rd_addr3]
  bus_expand2/3(out2) -> [rd_addr2]
  bus_expand2/1(msb_out4) -> [rd_addr0]
  bus_expand2/2(out3) -> [rd_addr1]
  Delay1/1 -> [rd_en0]
  Delay3/1 -> [rd_en1]
  Delay4/1 -> [rd_en2]
  Delay5/1 -> [rd_en3]
  Delay6/1 -> tge_rx_core0/1
  Delay7/1 -> tge_rx_core1/1
  Delay9/1 -> tge_rx_core2/1
  Delay11/1 -> tge_rx_core3/1
  tge_rx_core0/13 -> [vld_out0]
  tge_rx_core0/12 -> [tge_order_err0]
  tge_rx_core0/5 -> [lb_order_err0]
  tge_rx_core0/6 -> [max_buf0]
  tge_rx_core1/8 -> [rx_sync1]
  tge_rx_core1/1 -> [rx_dout1]
  tge_rx_core1/10 -> [tge_err1]
  tge_rx_core1/3 -> [lb_err1]
  tge_rx_core1/2 -> [lb_bad_addr1]
  tge_rx_core1/7 -> [mcnt_out1]
  tge_rx_core1/9 -> [tge_bad_addr1]
  tge_rx_core1/4 -> [lb_pkt_err1]
  tge_rx_core1/11 -> [tge_pkt_err1]
  tge_rx_core1/13 -> [vld_out1]
  tge_rx_core1/12 -> [tge_order_err1]
  tge_rx_core1/5 -> [lb_order_err1]
  tge_rx_core1/6 -> [max_buf1]
  tge_rx_core2/8 -> [rx_sync2]
  tge_rx_core2/1 -> [rx_dout2]
  tge_rx_core2/10 -> [tge_err2]
  tge_rx_core2/3 -> [lb_err2]
  tge_rx_core2/2 -> [lb_bad_addr2]
  tge_rx_core2/7 -> [mcnt_out2]
  tge_rx_core2/9 -> [tge_bad_addr2]
  tge_rx_core2/4 -> [lb_pkt_err2]
  tge_rx_core2/11 -> [tge_pkt_err2]
  tge_rx_core2/13 -> [vld_out2]
  tge_rx_core2/12 -> [tge_order_err2]
  tge_rx_core2/5 -> [lb_order_err2]
  tge_rx_core2/6 -> [max_buf2]
  tge_rx_core3/8 -> [rx_sync3]
  tge_rx_core3/1 -> [rx_dout3]
  tge_rx_core3/10 -> [tge_err3]
  tge_rx_core3/3 -> [lb_err3]
  tge_rx_core3/2 -> [lb_bad_addr3]
  tge_rx_core3/7 -> [mcnt_out3]
  tge_rx_core3/9 -> [tge_bad_addr3]
  tge_rx_core3/4 -> [lb_pkt_err3]
  tge_rx_core3/11 -> [tge_pkt_err3]
  tge_rx_core3/13 -> [vld_out3]
  tge_rx_core3/12 -> [tge_order_err3]
  tge_rx_core3/5 -> [lb_order_err3]
  tge_rx_core3/6 -> [max_buf3]
  ant_id1/1 -> [ant_id1]
  ctr_rst/1 -> [ctr_rst]
  [ctr_rst] -> Delay15/1
  [tge_bad_addr0] -> stats0/9(tge_bad_addr)
  [lb_err0] -> stats0/2(lb_err)
  [tge_order_err0] -> stats0/7(tge_order_err)
  [tge_err0] -> stats0/5(tge_err)
  [tge_pkt_err0] -> stats0/6(tge_pkt_err)
  [lb_order_err0] -> stats0/4(lb_order_err)
  [lb_bad_addr0] -> stats0/8(lb_bad_addr)
  [lb_pkt_err0] -> stats0/3(lb_pkt_err)
  [ctr_rst] -> Delay14/1
  [tge_bad_addr1] -> stats1/9(tge_bad_addr)
  [lb_err1] -> stats1/2(lb_err)
  [tge_order_err1] -> stats1/7(tge_order_err)
  [tge_err1] -> stats1/5(tge_err)
  [tge_pkt_err1] -> stats1/6(tge_pkt_err)
  [lb_order_err1] -> stats1/4(lb_order_err)
  [lb_bad_addr1] -> stats1/8(lb_bad_addr)
  [lb_pkt_err1] -> stats1/3(lb_pkt_err)
  [ctr_rst] -> Delay13/1
  [tge_bad_addr2] -> stats2/9(tge_bad_addr)
  [lb_err2] -> stats2/2(lb_err)
  [tge_order_err2] -> stats2/7(tge_order_err)
  [tge_err2] -> stats2/5(tge_err)
  [tge_pkt_err2] -> stats2/6(tge_pkt_err)
  [lb_order_err2] -> stats2/4(lb_order_err)
  [lb_bad_addr2] -> stats2/8(lb_bad_addr)
  [lb_pkt_err2] -> stats2/3(lb_pkt_err)
  [ctr_rst] -> Delay12/1
  [lb_bad_addr3] -> stats3/8(lb_bad_addr)
  [tge_err3] -> stats3/5(tge_err)
  [tge_bad_addr3] -> stats3/9(tge_bad_addr)
  [lb_err3] -> stats3/2(lb_err)
  [tge_order_err3] -> stats3/7(tge_order_err)
  [lb_order_err3] -> stats3/4(lb_order_err)
  [lb_pkt_err3] -> stats3/3(lb_pkt_err)
  [tge_pkt_err3] -> stats3/6(tge_pkt_err)
  Delay12/1 -> stats3/1(ctr_rst)
  Delay13/1 -> stats2/1(ctr_rst)
  Delay14/1 -> stats1/1(ctr_rst)
  Delay15/1 -> stats0/1(ctr_rst)
  sync1/1 -> [sync1]
  Delay16/1 -> xeng_packetiser0/3(mrst_in)
  Delay17/1 -> xeng_packetiser1/3(mrst_in)
  Delay18/1 -> xeng_packetiser2/3(mrst_in)
  Delay19/1 -> xeng_packetiser3/3(mrst_in)
  [gbe_enable0] -> Delay20/1
  Delay20/1 -> link1/7(gbe_en)
  masker1/1(dout) -> link2/1(tx_data)
  masker1/2(gbe_vld) -> link2/2(gbe_vld)
  masker1/3(ip_addr) -> link2/3(dest_ip)
  masker1/4(eof_out) -> link2/4(eof)
  masker1/5(lb_vld) -> link2/5(lb_vld)
  [mrst] -> link2/6(mrst)
  [gbe_enable0] -> Delay21/1
  Delay21/1 -> link2/7(gbe_en)
  masker2/1(dout) -> link3/1(tx_data)
  masker2/2(gbe_vld) -> link3/2(gbe_vld)
  masker2/3(ip_addr) -> link3/3(dest_ip)
  masker2/4(eof_out) -> link3/4(eof)
  masker2/5(lb_vld) -> link3/5(lb_vld)
  [mrst] -> link3/6(mrst)
  [gbe_enable1] -> Delay22/1
  Delay22/1 -> link3/7(gbe_en)
  masker3/2(gbe_vld) -> link4/2(gbe_vld)
  masker3/1(dout) -> link4/1(tx_data)
  masker3/3(ip_addr) -> link4/3(dest_ip)
  masker3/4(eof_out) -> link4/4(eof)
  masker3/5(lb_vld) -> link4/5(lb_vld)
  [mrst] -> link4/6(mrst)
  [gbe_enable1] -> Delay23/1
  Delay23/1 -> link4/7(gbe_en)
  gbe_en0/1 -> [gbe_enable0]
  gbe_en1/1 -> [gbe_enable1]
